simulink model "SecondOrderSystemAdjustment_UnstableSystem"  (R2013b)
settings: Solver=ode45  StartTime=0.0  StopTime=15  RelTol=1e-3
settings Model: Creator=MMSA  LastModifiedBy=MMSA
settings SolverCC: MaxConsecutiveZCs=1  ZeroCrossAlgorithm=Adaptive  PositivePriorityOrder=on
settings DataIOCC: LimitDataPoints=off  SaveOutput=off
settings HardwareCC: ProdBitPerPointer=64  ProdHWDeviceType=Generic->64-bit Embedded Processor (LLP64)

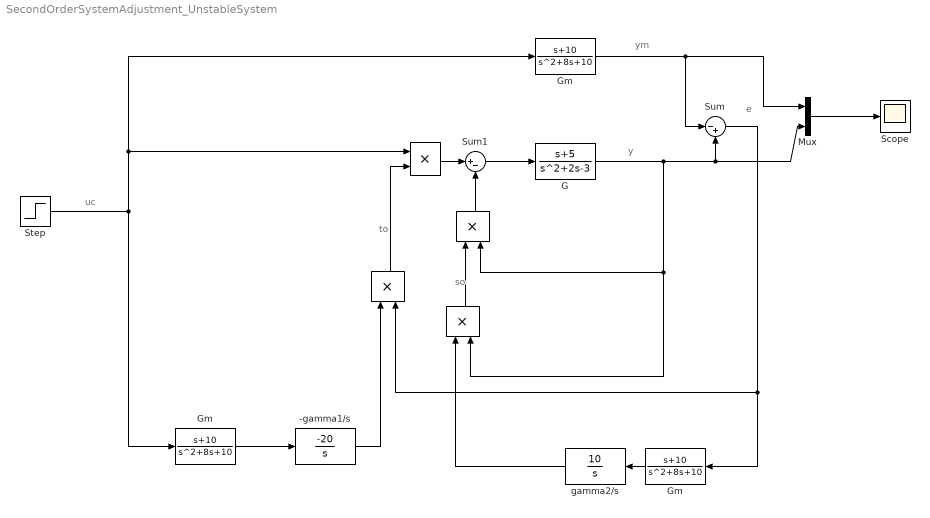
== system SecondOrderSystemAdjustment_UnstableSystem ==
  note: e
  note: so
  note: to
  note: uc
  note: ym
  note: y
  " " : Product
  " " : Product
  "  " : Product
  "     " : Product
  -gamma1/s : TransferFcn  Numerator=[-20]  Denominator=[1 0]
  G : TransferFcn  Numerator=[1 5]  Denominator=[1 2 -3]
  Gm : TransferFcn  Numerator=[1 10]  Denominator=[1 8 10]
  "Gm " : TransferFcn  Numerator=[1 10]  Denominator=[1 8 10]
  "Gm  " : TransferFcn  Numerator=[1 10]  Denominator=[1 8 10]
  Mux : Mux  Inputs=2
  Scope : Scope
      settings: TimeRange=30  YMin=-1.883072367020043e-70  YMax=1
  Step : Step  Time=0  SampleTime=0
  Sum : Sum  Inputs=|-+
  Sum1 : Sum  Inputs=|+-
  gamma2/s : TransferFcn  Numerator=[10]  Denominator=[1 0]
  wires:
  Mux/1 -> Scope/1
  Gm/1 -> Sum/1, Mux/1
  Step/1 -> "Gm  "/1, Gm/1, "     "/1
  G/1 -> Sum/2, Mux/2, " "/2, "  "/2
  Sum/1 -> " "/2, "Gm "/1
  -gamma1/s/1 -> " "/1
  Sum1/1 -> G/1
  "Gm  "/1 -> -gamma1/s/1
  "Gm "/1 -> gamma2/s/1
  gamma2/s/1 -> "  "/1
  "  "/1 -> " "/1
  " "/1 -> Sum1/2
  "     "/1 -> Sum1/1
  " "/1 -> "     "/2
